simulink model "single_phase_half_wave_rectifier"  (R2024b)
settings: Solver=ode4  StartTime=0.0  StopTime=4/50  FixedStep=10e-6  RelTol=1e-3
libraries: spsVoltageMeasurementLib x3, spsSeriesRLCBranchLib x3, spsACVoltageSourceLib x2, spsDiodeLib x2, spspowerguiLib x1
settings Model: Creator=Abhijith_Kumble  LastModifiedBy=Abhijith_Kumble

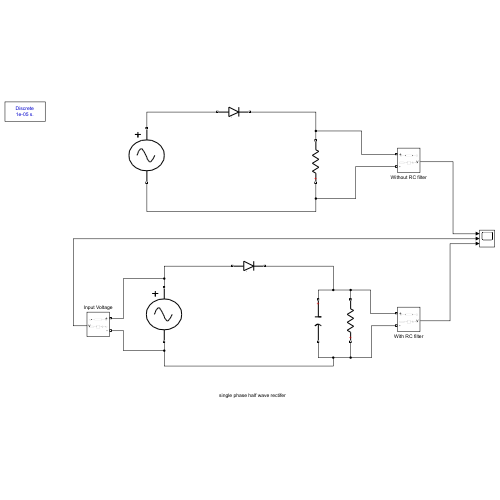
[thumbnail: Simulink's stored preview of the top-level diagram]
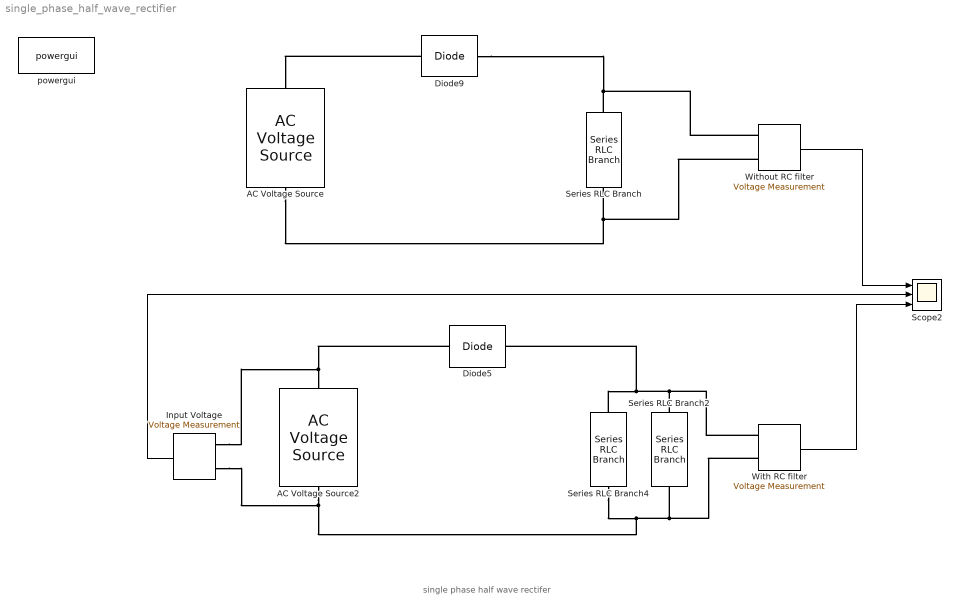
== system single_phase_half_wave_rectifier ==
  note: single phase half wave rectifer
  AC Voltage Source : spsACVoltageSourceLib/AC Voltage Source  Amplitude=230  Phase=0  Frequency=50  SampleTime=0  Measurements=None  BusType=swing  Pref=10e3  Qref=0  Qmin=-inf  Qmax=+inf
  AC Voltage Source2 : spsACVoltageSourceLib/AC Voltage Source  Amplitude=230  Phase=0  Frequency=50  SampleTime=0  Measurements=None  BusType=swing  Pref=10e3  Qref=0  Qmin=-inf  Qmax=+inf
  Diode5 : spsDiodeLib/Diode  Ron=0.001  Lon=0  Vf=0.0  IC=0  UseSnubber=0  Rs=0  Cs=0  Measurements=off
  Diode9 : spsDiodeLib/Diode  Ron=0.001  Lon=0  Vf=0.0  IC=0  UseSnubber=0  Rs=0  Cs=0  Measurements=off
  Input Voltage : spsVoltageMeasurementLib/Voltage Measurement  PhasorSimulation=off  OutputType=Complex  PSBequivalent=0
  Scope2 : Scope  NumInputPorts=3
  Series RLC Branch : spsSeriesRLCBranchLib/Series RLC Branch  LConnTagsString=__new0  RConnTagsString=__new0  BranchType=R  Resistance=1  Inductance=1e-3  SetiL0=off  InitialCurrent=0  Capacitance=1e-6  Setx0=off  InitialVoltage=0  Measurements=None
  Series RLC Branch2 : spsSeriesRLCBranchLib/Series RLC Branch  LConnTagsString=__new0  RConnTagsString=__new0  BranchType=R  Resistance=1000  Inductance=1e-3  SetiL0=off  InitialCurrent=0  Capacitance=1e-6  Setx0=off  InitialVoltage=0  Measurements=None
  Series RLC Branch4 : spsSeriesRLCBranchLib/Series RLC Branch  LConnTagsString=__new0  RConnTagsString=__new0  BranchType=C  Resistance=1  Inductance=1e-3  SetiL0=off  InitialCurrent=0  Capacitance=100*10e-6  Setx0=off  InitialVoltage=0  Measurements=None
  With RC filter : spsVoltageMeasurementLib/Voltage Measurement  PhasorSimulation=off  OutputType=Complex  PSBequivalent=0
  Without RC filter : spsVoltageMeasurementLib/Voltage Measurement  PhasorSimulation=off  OutputType=Complex  PSBequivalent=0
  powergui : spspowerguiLib/powergui  Priority=1  SimulationMode=Discrete  SampleTime=10e-6  frequency=50  Iterations=50  frequencyindice=50  Pbase=100e6  ErrMax=1e-4  UnitsV=kV  UnitsW=MW  buscounter=0  FunctionMessages=off  echomessages=off  EnableUseOfTLC=off  CurrentSourceSwitches=off  DisableSnubberDevices=off  DisableRonSwitches=off  DisableVfSwitches=off  DisplayEquations=off  AutomaticDiscreteSolvers=off  SolverType=Tustin/Backward Euler (TBE)  Interpol=off  ExternalGateDelay=off  methode=off  Ts=100  x0status=blocks  SPID=on  SwTol=0  HookPort=off  NonlinearTolerance=1e-4  nMaxIteration=100  ContinueOnMaxIteration=off  RestoreLinks=warning  ResistiveCurrentMeasurement=off  Frange=[0:2:500]  Ylog=off  Xlog=on  ShowGrid=off  save=off  variable=ZData  structure=0  ZoomFFT=off  StartTime=0.0  cycles=1  DisplayStyle=1  fundamental=60  FreqAxis=off  MaxFrequency=1000  frequencyindicesteady=1  RmsSteady=1  display=off
  wires:
  Without RC filter/1 -> Scope2/1
  Input Voltage/1 -> Scope2/2
  With RC filter/1 -> Scope2/3
  connections:
  Without RC filter/LConn1 -- Diode9/RConn1 -- Series RLC Branch/RConn1
  Diode5/LConn1 -- Input Voltage/LConn1 -- AC Voltage Source2/RConn1
  Series RLC Branch/LConn1 -- AC Voltage Source/LConn1 -- Without RC filter/LConn2
  Series RLC Branch2/RConn1 -- With RC filter/LConn1 -- Series RLC Branch4/LConn1 -- Diode5/RConn1
  With RC filter/LConn2 -- Series RLC Branch2/LConn1 -- Input Voltage/LConn2 -- AC Voltage Source2/LConn1 -- Series RLC Branch4/RConn1
  Diode9/LConn1 -- AC Voltage Source/RConn1
